simulink model "DoublePulseTestSLX"  (R2016a)
settings: Solver=FixedStepDiscrete  StartTime=0.0  StopTime=25e-6  FixedStep=SampleTime  RelTol=1e-3
values from neighbouring files (symbols this model uses):
  Dbot = 19    [DoublePulseTestM.m]
  DelayBot = 50    [DoublePulseTestM.m]
  DelayTop = 0    [DoublePulseTestM.m]
  Dtop = 19    [DoublePulseTestM.m]
  fsw = 20e3    (= 20000)    [DoublePulseTestM.m]
  Lload = 250e-6    (= 0.00025)    [DoublePulseTestM.m]
  LoadCurrent = 30    [DoublePulseTestM.m]
  SampleTime = 1e-9    (= 1e-09)    [DoublePulseTestM.m]
  Vdc = 400    [DoublePulseTestM.m]
  VpulseMax = 6    [DoublePulseTestM.m]
  VpulseMin = 0    [DoublePulseTestM.m]
libraries: fl_lib x12, nesl_utility x10, elec_lib x4, pe_lib x2
settings Model: Creator=ugurm  LastModifiedBy=Furkan
settings OptimizationCC: EfficientMapNaN2IntZero=off
settings HardwareCC: TargetBitPerPointer=64  TargetLongLongMode=on  TargetIntDivRoundTo=Zero  TargetEndianess=LittleEndian  TargetWordSize=64  TargetHWDeviceType=MATLAB Host  ProdEqTarget=off
settings CodeAppCC: MaxIdLength=128
settings GRTTargetCC: GeneratePreprocessorConditionals=Use local settings  CombineOutputUpdateFcns=off  GRTInterface=on

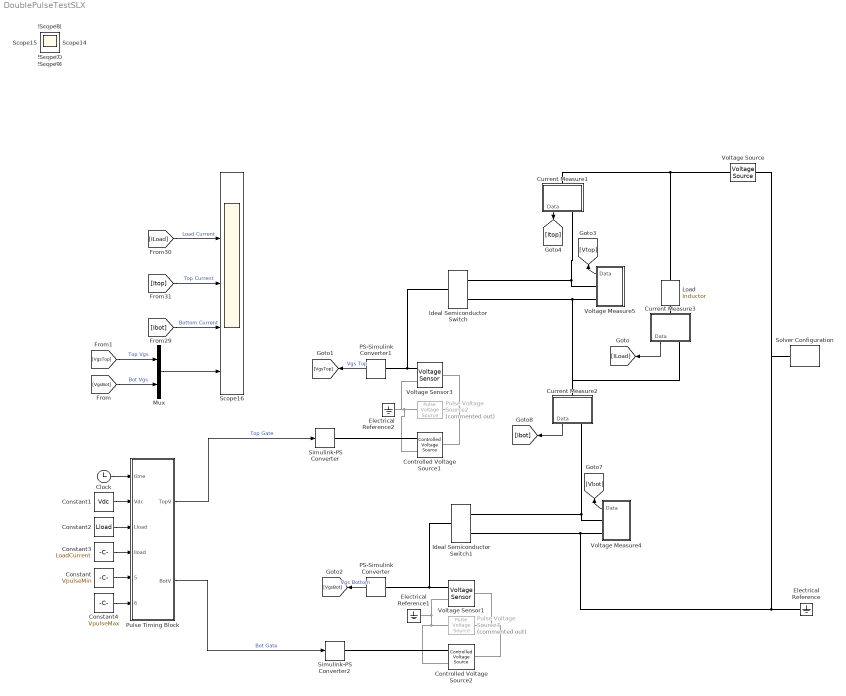
== system DoublePulseTestSLX ==
  Clock : Clock
  Constant : Constant  Value=VpulseMin
  Constant1 : Constant  Value=Vdc
  Constant2 : Constant  Value=Lload
  Constant3 : Constant  Value=LoadCurrent
  Constant4 : Constant  Value=VpulseMax
  Controlled Voltage Source1 : fl_lib/Electrical/Electrical Sources/Controlled Voltage Source
  Controlled Voltage Source2 : fl_lib/Electrical/Electrical Sources/Controlled Voltage Source
  Current Measure1 : Subsystem
  Current Measure2 : Subsystem
  Current Measure3 : Subsystem
  Electrical Reference : fl_lib/Electrical/Electrical Elements/Electrical Reference
  Electrical Reference1 : fl_lib/Electrical/Electrical Elements/Electrical Reference
  Electrical Reference2 : fl_lib/Electrical/Electrical Elements/Electrical Reference
  Ideal Semiconductor Switch : pe_lib/Semiconductors/Fundamental Components/Ideal Semiconductor Switch  Ron=0.001 Ohm  Goff=1e-6 1/Ohm  Vth=0.5 V  diode_param=2  diode_Vf=0.8 V  diode_Ron=0.001 Ohm  diode_Goff=1e-5 1/Ohm  diode_C=5e-8 F  diode_iRM=-235 A  diode_iF=300 A  diode_idot=-50 A/us  diode_trr_param=1  diode_trr_factor=3  diode_trr=15 us  diode_Qrr=1.5e+3 s*uA
  Ideal Semiconductor Switch1 : pe_lib/Semiconductors/Fundamental Components/Ideal Semiconductor Switch  Ron=0.001 Ohm  Goff=1e-6 1/Ohm  Vth=0.5 V  diode_param=2  diode_Vf=0.8 V  diode_Ron=0.001 Ohm  diode_Goff=1e-5 1/Ohm  diode_C=5e-8 F  diode_iRM=-235 A  diode_iF=300 A  diode_idot=-50 A/us  diode_trr_param=1  diode_trr_factor=3  diode_trr=15 us  diode_Qrr=1.5e+3 s*uA
  Load : elec_lib/Passive Devices/Inductor  l=Lload H  L_tol=20  enable_L_tol=0  tol_distribution=1  nSigma=4  r=0 Ohm  g=1e-9 1/Ohm  initI=InitialCurrent A  enable_operating_limits=0  operating_limit_action=2  max_working_current=1 A  power_rating=1 W  enable_faults=0  fault_action=1  lambdaPercent=50  k_faulted=0.9999 Ohm  turnsShort=0  openCct=0  groundShort=0  groundShortG=0 1/Ohm  tau_fault=0.001 s  enable_temporal_fault=0  t_fault=1 s  enable_behavioral_fault=0  max_permissible_voltage=100 V  n_fail_on_voltage=1  max_permissible_current=1 A  t_fail_on_current=1 s
  Mux : Mux  Inputs=2
  PS-Simulink Converter : nesl_utility/PS-Simulink Converter  PhysicalDomain=network_engine_domain  SubClassName=ps_output  LeftPortType=input  RightPortType=output  PseudoPeriodic=off  Frequencies=[]  Unit=1  AffineConversion=off
  PS-Simulink Converter1 : nesl_utility/PS-Simulink Converter  PhysicalDomain=network_engine_domain  SubClassName=ps_output  LeftPortType=input  RightPortType=output  PseudoPeriodic=off  Frequencies=[]  Unit=1  AffineConversion=off
  Pulse Timing Block : MATLAB Function  TreatAsAtomicUnit=on  SystemSampleTime=SampleTime
  Pulse Voltage Source2 : elec_lib/Additional Components/SPICE-Compatible Components/Sources/Pulse Voltage Source  Commented=on  V1=VpulseMin V  V2=VpulseMax V  TD=DelayTop/(100*fsw) s  TR=1e-9 s  TF=1e-9 s  PW=Dtop/(100*fsw) s  PER=1/fsw s
  Pulse Voltage Source3 : elec_lib/Additional Components/SPICE-Compatible Components/Sources/Pulse Voltage Source  Commented=on  V1=VpulseMin V  V2=VpulseMax V  TD=DelayBot/(100*fsw) s  TR=1e-9 s  TF=1e-9 s  PW=Dbot/(100*fsw) s  PER=1/fsw s
  Scope16 : Scope  NumInputPorts=5
  Simulink-PS Converter : nesl_utility/Simulink-PS Converter  PhysicalDomain=network_engine_domain  SubClassName=ps_input  LeftPortType=input  RightPortType=output  PseudoPeriodic=off  Frequencies=[]  NoiseDistribution=none  NoiseParameters=[]  Unit=1  AffineConversion=off  InputFiltering=off  SimscapeFilterOrder=1  InputFilterTimeConstant=0.001  UdotUserProvided=1
  Simulink-PS Converter2 : nesl_utility/Simulink-PS Converter  PhysicalDomain=network_engine_domain  SubClassName=ps_input  LeftPortType=input  RightPortType=output  PseudoPeriodic=off  Frequencies=[]  NoiseDistribution=none  NoiseParameters=[]  Unit=1  AffineConversion=off  InputFiltering=off  SimscapeFilterOrder=1  InputFilterTimeConstant=0.001  UdotUserProvided=1
  Solver Configuration : nesl_utility/Solver Configuration  PhysicalDomain=network_engine_domain  SubClassName=solver  LeftPortType=input  RightPortType=generic  Accelerate=off  Tones=[]  Harmonics=[]  SimulateNoise=off  Profile=off  UseLocalSampling=off  EnableSwitchedLinearOptims=on  FrequencyDomain=off  UseCCode=off  RelTol=0.001  AbsTol=1e-06  MinStep=1e-09  ToWorkspace=off  RevertToSquareIcSolve=off  NumHomotopyIterations=100  PhasorMode=off  PhasorModeNumHarmonics=1  OverrideAbsTol=off  DoDC=off  ResidualTolerance=1e-09  UseLocalSolver=on  LocalSolverChoice=NE_BACKWARD_EULER_ADVANCER  LocalSolverSampleTime=SampleTime  DoFixedCost=on  MaxNonlinIter=3  MaxModeIter=2  LinearAlgebra=Sparse  DelaysMemoryBudget=1024  AutomaticFiltering=on  FilteringTimeConstant=0.001
  Voltage Measure4 : Subsystem
  Voltage Measure5 : Subsystem
  Voltage Sensor1 : fl_lib/Electrical/Electrical Sensors/Voltage Sensor
  Voltage Sensor3 : fl_lib/Electrical/Electrical Sensors/Voltage Sensor
  Voltage Source : elec_lib/Sources/Voltage Source  dc_voltage=Vdc V  ac_voltage=0 V  ac_shift=0 deg  ac_frequency=60 Hz  noise_mode=0  PSD=0 V^2/Hz  sample_time=0.001 s  repeatability=1  auto_seed=545404223  user_seed=0
  Scope{7..11,13..15} (8 alike) : Scope
  wires:
  Current Measure3/1(Data) -> [ILoad]
  Voltage Measure4/1(Data) -> [Vbot]
  Voltage Measure5/1(Data) -> [Vtop]
  Current Measure1/1(Data) -> [Itop]
  [Ibot] -> Scope16/4  "Bottom Current"
  [Itop] -> Scope16/3  "Top Current"
  [ILoad] -> Scope16/2  "Load Current"
  Clock/1 -> Pulse Timing Block/1(time)
  Pulse Timing Block/1(TopV) -> Simulink-PS Converter/1  "Top Gate"
  Pulse Timing Block/2(BotV) -> Simulink-PS Converter2/1  "Bot Gate"
  Mux/1 -> Scope16/5
  Current Measure2/1(Data) -> [Ibot]
  PS-Simulink Converter1/1 -> [VgsTop]  "Vgs Top"
  PS-Simulink Converter/1 -> [VgsBot]  "Vgs Bottom"
  [VgsBot] -> Mux/2  "Bot Vgs"
  [VgsTop] -> Mux/1  "Top Vgs"
  Constant1/1 -> Pulse Timing Block/2(Vdc)
  Constant2/1 -> Pulse Timing Block/3(Lload)
  Constant3/1 -> Pulse Timing Block/4(Iload)
  Constant/1 -> Pulse Timing Block/5(VpulseMin)
  Constant4/1 -> Pulse Timing Block/6(VpulseMax)
  connections:
  Ideal Semiconductor Switch/RConn1 -- Current Measure1/RConn1 -- Voltage Measure5/RConn1
  Current Measure1/LConn1 -- Load/LConn1 -- Voltage Source/LConn1
  Ideal Semiconductor Switch1/RConn2 -- Electrical Reference/LConn1 -- Voltage Source/RConn1 -- Solver Configuration/RConn1 -- Voltage Measure4/RConn2
  Pulse Voltage Source2/RConn1 -- Controlled Voltage Source1/RConn2 -- Voltage Sensor3/RConn2 -- Electrical Reference2/LConn1
  Pulse Voltage Source2/LConn1 -- Controlled Voltage Source1/LConn1 -- Voltage Sensor3/LConn1
  Voltage Sensor3/RConn1 -- Ideal Semiconductor Switch/LConn1 -- PS-Simulink Converter1/LConn1
  Pulse Voltage Source3/LConn1 -- Controlled Voltage Source2/LConn1 -- Voltage Sensor1/LConn1
  Pulse Voltage Source3/RConn1 -- Controlled Voltage Source2/RConn2 -- Electrical Reference1/LConn1 -- Voltage Sensor1/RConn2
  Voltage Sensor1/RConn1 -- Ideal Semiconductor Switch1/LConn1 -- PS-Simulink Converter/LConn1
  Simulink-PS Converter/RConn1 -- Controlled Voltage Source1/RConn1
  Simulink-PS Converter2/RConn1 -- Controlled Voltage Source2/RConn1
  Voltage Measure5/RConn2 -- Current Measure3/RConn1 -- Current Measure2/LConn1 -- Ideal Semiconductor Switch/RConn2
  Ideal Semiconductor Switch1/RConn1 -- Voltage Measure4/RConn1 -- Current Measure2/RConn1
  Current Measure3/LConn1 -- Load/RConn1

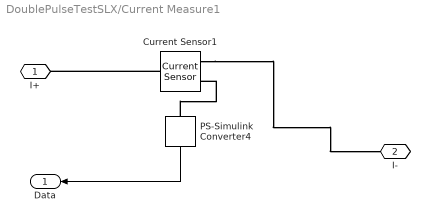
== system DoublePulseTestSLX/Current Measure1 ==
  Current Sensor1 : fl_lib/Electrical/Electrical Sensors/Current Sensor
  PS-Simulink Converter4 : nesl_utility/PS-Simulink Converter  PhysicalDomain=network_engine_domain  SubClassName=ps_output  LeftPortType=input  RightPortType=output  PseudoPeriodic=off  Frequencies=[]  Unit=1  AffineConversion=off
  I+ : PMIOPort  Port=1  Side=Left
  I- : PMIOPort  Port=2  Side=Right
  Data : Outport
  wires:
  PS-Simulink Converter4/1 -> Data/1
  connections:
  Current Sensor1/RConn2 -- I-/RConn1
  PS-Simulink Converter4/LConn1 -- Current Sensor1/RConn1
  Current Sensor1/LConn1 -- I+/RConn1

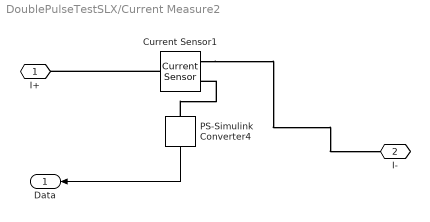
== system DoublePulseTestSLX/Current Measure2 ==
  Current Sensor1 : fl_lib/Electrical/Electrical Sensors/Current Sensor
  PS-Simulink Converter4 : nesl_utility/PS-Simulink Converter  PhysicalDomain=network_engine_domain  SubClassName=ps_output  LeftPortType=input  RightPortType=output  PseudoPeriodic=off  Frequencies=[]  Unit=1  AffineConversion=off
  I+ : PMIOPort  Port=1  Side=Left
  I- : PMIOPort  Port=2  Side=Right
  Data : Outport
  wires:
  PS-Simulink Converter4/1 -> Data/1
  connections:
  Current Sensor1/RConn2 -- I-/RConn1
  PS-Simulink Converter4/LConn1 -- Current Sensor1/RConn1
  Current Sensor1/LConn1 -- I+/RConn1

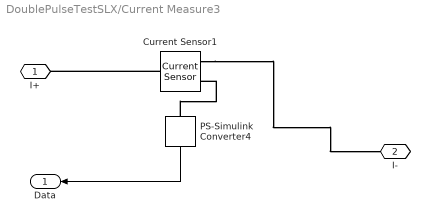
== system DoublePulseTestSLX/Current Measure3 ==
  Current Sensor1 : fl_lib/Electrical/Electrical Sensors/Current Sensor
  PS-Simulink Converter4 : nesl_utility/PS-Simulink Converter  PhysicalDomain=network_engine_domain  SubClassName=ps_output  LeftPortType=input  RightPortType=output  PseudoPeriodic=off  Frequencies=[]  Unit=1  AffineConversion=off
  I+ : PMIOPort  Port=1  Side=Left
  I- : PMIOPort  Port=2  Side=Right
  Data : Outport
  wires:
  PS-Simulink Converter4/1 -> Data/1
  connections:
  Current Sensor1/LConn1 -- I+/RConn1
  PS-Simulink Converter4/LConn1 -- Current Sensor1/RConn1
  Current Sensor1/RConn2 -- I-/RConn1

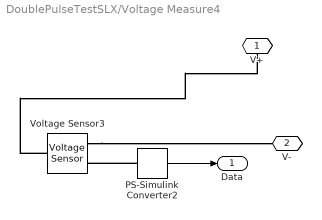
== system DoublePulseTestSLX/Voltage Measure4 ==
  PS-Simulink Converter2 : nesl_utility/PS-Simulink Converter  PhysicalDomain=network_engine_domain  SubClassName=ps_output  LeftPortType=input  RightPortType=output  PseudoPeriodic=off  Frequencies=[]  Unit=1  AffineConversion=off
  Voltage Sensor3 : fl_lib/Electrical/Electrical Sensors/Voltage Sensor
  V+ : PMIOPort  Port=1  Side=Right
  V- : PMIOPort  Port=2  Side=Right
  Data : Outport
  wires:
  PS-Simulink Converter2/1 -> Data/1
  connections:
  Voltage Sensor3/LConn1 -- V+/RConn1
  Voltage Sensor3/RConn2 -- V-/RConn1
  PS-Simulink Converter2/LConn1 -- Voltage Sensor3/RConn1

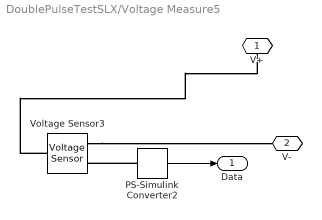
== system DoublePulseTestSLX/Voltage Measure5 ==
  PS-Simulink Converter2 : nesl_utility/PS-Simulink Converter  PhysicalDomain=network_engine_domain  SubClassName=ps_output  LeftPortType=input  RightPortType=output  PseudoPeriodic=off  Frequencies=[]  Unit=1  AffineConversion=off
  Voltage Sensor3 : fl_lib/Electrical/Electrical Sensors/Voltage Sensor
  V+ : PMIOPort  Port=1  Side=Right
  V- : PMIOPort  Port=2  Side=Right
  Data : Outport
  wires:
  PS-Simulink Converter2/1 -> Data/1
  connections:
  PS-Simulink Converter2/LConn1 -- Voltage Sensor3/RConn1
  Voltage Sensor3/RConn2 -- V-/RConn1
  Voltage Sensor3/LConn1 -- V+/RConn1

== matlab function DoublePulseTestSLX/Pulse Timing Block ==
  data: TopV output; BotV output; time input; Vdc input; Lload input; Iload input; VpulseMin input; VpulseMax input
function [TopV,BotV]= fcn(time,Vdc,Lload,Iload,VpulseMin,VpulseMax)
ChargeTime = Lload * Iload / Vdc;
DeadTime = 100e-9;
GapTime = 5e-6;
if time <= ChargeTime
    BotV = VpulseMax;
    TopV = VpulseMin;
elseif time <= (ChargeTime + DeadTime)
    BotV = VpulseMin;
    TopV = VpulseMin;
elseif time <= (ChargeTime + GapTime)
    BotV = VpulseMin;
    TopV = VpulseMax;
elseif time <= (ChargeTime + GapTime + DeadTime)
    BotV = VpulseMin;
    TopV = VpulseMin;
elseif time <= (ChargeTime + GapTime + DeadTime + DeadTime)
    BotV = VpulseMax;
    TopV = VpulseMin;
else
    BotV = VpulseMin;
    TopV = VpulseMin;
end
